simulink model "roachf_1024_bao"  (Simulink 7.5)
settings: Solver=ode45  StartTime=0.0  StopTime=10.0  RelTol=1e-3
undefined symbols (not defined in the file or in its folder): Down, quant, Up
libraries: xbsIndex_r4 x1081, xps_library x49, casper_library_misc x17, casper_library_delays x9, casper_library_sources x4, xbsReplacements_r4 x4, xrbsControl_r4 x1
(part 2 of 11)

== system roachf_1024_bao/status ==
  Concat : xbsIndex_r4/Concat  num_inputs=8  dbl_ovrd=off  block_type=concat
  Concat1 : xbsIndex_r4/Concat  num_inputs=8  dbl_ovrd=off  block_type=concat
  Constant1 : xbsIndex_r4/Constant  const=0  gui_display_data_type=Fixed-point  arith_type=Unsigned  n_bits=25  bin_pt=0  preci_type=Single  exp_width=8  frac_width=24  explicit_period=on  period=1  equ=P=C  opselect=C  inp2=PCIN>>17  opr=+  inp1=P  carry=CIN  dbl_ovrd=off  block_type=constant
      settings: block_version=11.4
  Constant2 : xbsIndex_r4/Constant  const=0  gui_display_data_type=Fixed-point  arith_type=Unsigned  n_bits=25  bin_pt=0  preci_type=Single  exp_width=8  frac_width=24  explicit_period=on  period=1  equ=P=C  opselect=C  inp2=PCIN>>17  opr=+  inp1=P  carry=CIN  dbl_ovrd=off  block_type=constant
      settings: block_version=11.4
  Counter1 : xbsIndex_r4/Counter  cnt_type=Free Running  cnt_to=Inf  operation=Up  start_count=0  cnt_by_val=1  arith_type=Unsigned  n_bits=32  bin_pt=0  load_pin=off  rst=on  en=on  explicit_period=on  period=1  dbl_ovrd=off  use_behavioral_HDL=off  implementation=Fabric  block_type=counter
  Counter2 : xbsIndex_r4/Counter  cnt_type=Free Running  cnt_to=Inf  operation=Up  start_count=0  cnt_by_val=1  arith_type=Unsigned  n_bits=32  bin_pt=0  load_pin=off  rst=on  en=on  explicit_period=on  period=1  dbl_ovrd=off  use_behavioral_HDL=off  implementation=Fabric  block_type=counter
  Counter3 : xbsIndex_r4/Counter  cnt_type=Free Running  cnt_to=Inf  operation=Up  start_count=0  cnt_by_val=1  arith_type=Unsigned  n_bits=32  bin_pt=0  load_pin=off  rst=on  en=on  explicit_period=on  period=1  dbl_ovrd=off  use_behavioral_HDL=off  implementation=Fabric  block_type=counter
  gbe_gpu : xps_library/software register  Tag=xps:sw_reg  SystemSampleTime=-1  io_dir=To Processor  arith_type=Unsigned  bitwidth=32  bin_pt=0  sample_period=1  gw_name=roachf_1024_bao_status_gbe_gpu_user_data_in
  gbe_sw : xps_library/software register  Tag=xps:sw_reg  SystemSampleTime=-1  io_dir=To Processor  arith_type=Unsigned  bitwidth=32  bin_pt=0  sample_period=1  gw_name=roachf_1024_bao_status_gbe_sw_user_data_in
  swgbe_bframe : xps_library/software register  Tag=xps:sw_reg  SystemSampleTime=-1  io_dir=To Processor  arith_type=Unsigned  bitwidth=32  bin_pt=0  sample_period=1  gw_name=roachf_1024_bao_status_swgbe_bframe_user_data_in
      link override convert: arith_type=Unsigned  n_bits=32  bin_pt=0
  swgbe_oflow : xps_library/software register  Tag=xps:sw_reg  SystemSampleTime=-1  io_dir=To Processor  arith_type=Unsigned  bitwidth=32  bin_pt=0  sample_period=1  gw_name=roachf_1024_bao_status_swgbe_oflow_user_data_in
      link override convert: arith_type=Unsigned  n_bits=32  bin_pt=0
  swgbe_orun : xps_library/software register  Tag=xps:sw_reg  SystemSampleTime=-1  io_dir=To Processor  arith_type=Unsigned  bitwidth=32  bin_pt=0  sample_period=1  gw_name=roachf_1024_bao_status_swgbe_orun_user_data_in
      link override convert: arith_type=Unsigned  n_bits=32  bin_pt=0
  wires:
  Concat/1 -> gbe_sw/1
  Constant1/1 -> Concat/1
  [gbe_sw_led_up] -> Concat/2
  [gbe_sw_led_rx] -> Concat/3
  [gbe_sw_led_tx] -> Concat/4
  [gbe_sw_tx_afull] -> Concat/5
  [gbe_sw_tx_oflow] -> Concat/6
  [gbe_sw_rx_bfr] -> Concat/7
  [gbe_sw_rx_orun] -> Concat/8
  Concat1/1 -> gbe_gpu/1
  Constant2/1 -> Concat1/1
  [gbe_gpu_led_up] -> Concat1/2
  [gbe_gpu_led_rx] -> Concat1/3
  [gbe_gpu_led_tx] -> Concat1/4
  [gbe_gpu_tx_ack] -> Concat1/5
  [gbe_gpu_rx_valid] -> Concat1/6
  [gbe_gpu_rx_eof] -> Concat1/7
  [gbe_gpu_rx_eof] -> Concat1/8
  Counter2/1 -> swgbe_bframe/1
  [gbe_sw_rx_bfr] -> Counter2/2
  [cnt_rst] -> Counter2/1
  Counter1/1 -> swgbe_orun/1
  [gbe_sw_rx_orun] -> Counter1/2
  [cnt_rst] -> Counter1/1
  Counter3/1 -> swgbe_oflow/1
  [gbe_sw_tx_oflow] -> Counter3/2
  [cnt_rst] -> Counter3/1

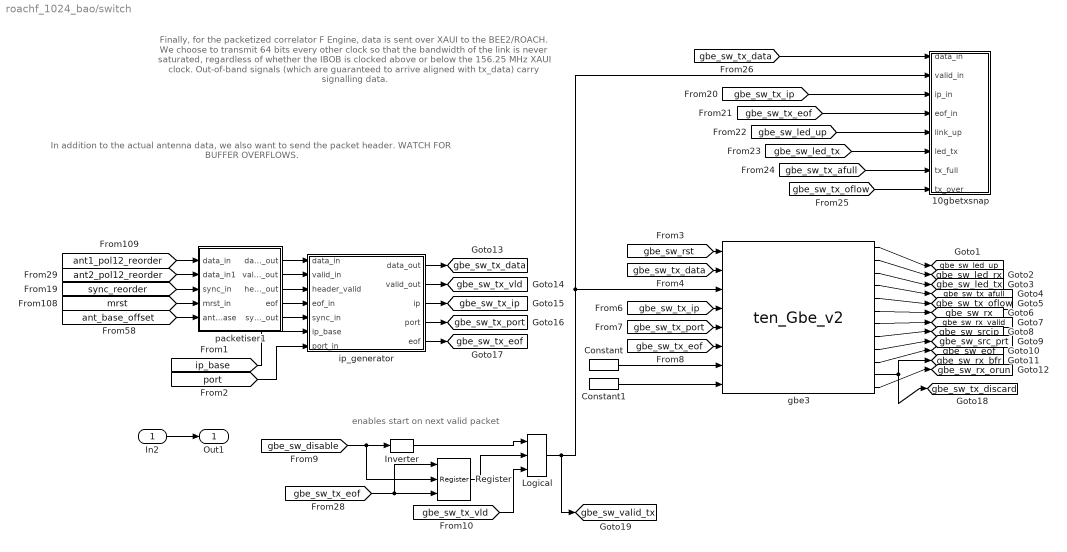
== system roachf_1024_bao/switch ==
  note: Finally, for the packetized correlator F Engine, data is sent over
      | XAUI to the BEE2/ROACH.  We choose to transmit 64 bits every other clock
      | so that the bandwidth of the link is never saturated, regardless of whether
      | the IBOB is clocked above or below the 156.25 MHz XAUI clock.
      | Out-of-band signals (which are guaranteed to arrive aligned with
      | tx_data) carry signalling data.
  note: In addition to the actual antenna data,
      | we also want to send the packet header.
      | WATCH FOR BUFFER OVERFLOWS.
  note: enables start on next valid packet
  In2 : Inport
  10gbetxsnap : Subsystem  mask{nsamples=10}
      mask prompts: nsamples "Number of samples (2^?)"
  Constant : xbsIndex_r4/Constant  const=1  gui_display_data_type=Fixed-point  arith_type=Boolean  n_bits=16  bin_pt=14  preci_type=Single  exp_width=8  frac_width=24  explicit_period=on  period=1  equ=P=C  opselect=C  inp2=PCIN>>17  opr=+  inp1=P  carry=CIN  dbl_ovrd=off  block_type=constant
      settings: block_version=11.4
  Constant1 : xbsIndex_r4/Constant  const=0  gui_display_data_type=Fixed-point  arith_type=Boolean  n_bits=16  bin_pt=14  preci_type=Single  exp_width=8  frac_width=24  explicit_period=on  period=1  equ=P=C  opselect=C  inp2=PCIN>>17  opr=+  inp1=P  carry=CIN  dbl_ovrd=off  block_type=constant
      settings: block_version=11.4
  Inverter : xbsIndex_r4/Inverter  en=off  latency=0  dbl_ovrd=off  block_type=inv
      settings: block_version=11.4
  Logical : xbsIndex_r4/Logical  logical_function=AND  inputs=3  en=off  latency=0  precision=Full  arith_type=Unsigned  n_bits=16  bin_pt=0  align_bp=on  dbl_ovrd=off  block_type=logical
      settings: block_version=11.4
  Register : xbsIndex_r4/Register  init=0  rst=on  en=on  dbl_ovrd=off  block_type=register
  gbe3 : xps_library/ten_Gbe_v2  Tag=xps:tengbe_v2  SystemSampleTime=-1  port=3  rx_dist_ram=off  large_frames=on  show_param=off  pre_emph=3  swing=800  fab_en=off  fab_mac=hex2dec('123456780000')  fab_ip=192*(2^24) + 168*(2^16) + 5*(2^8) + 20*(2^0)  fab_udp=10000  fab_gate=1  cpu_rx_en=on  cpu_tx_en=on
  ip_generator : Subsystem
  packetiser1 : Subsystem  mask{nwrd_bits=10, ant_bits=1, nSpec=4, nXeng=3, nChan=10}
      mask prompts: nwrd_bits "Payload length: (in 64bit words) (2^n)"; ant_bits "Number of antennas on this link (2^n)"; nSpec "Number of spectra(time samples) to acc. (2^?)"; nXeng "Number of Xengines total (2^?)"; nChan "Number of Channels in a spectra(2^?)"
      mask help: Wideband packetiser. Package 32 bit data into 64 bits and identify data as coming from antenna 0 or 1.
  Out1 : Outport
  tag scope: gbe_sw_eof=global, gbe_sw_led_rx=global, gbe_sw_led_tx=global, gbe_sw_led_up=global, gbe_sw_rx=global, gbe_sw_rx_bfr=global, gbe_sw_rx_orun=global, gbe_sw_rx_valid=global, gbe_sw_src_prt=global, gbe_sw_srcip=global, gbe_sw_tx_afull=global, gbe_sw_tx_data=global, gbe_sw_tx_discard=global, gbe_sw_tx_eof=global, gbe_sw_tx_ip=global, gbe_sw_tx_oflow=global, gbe_sw_tx_port=global, gbe_sw_tx_vld=global, gbe_sw_valid_tx=global
  wires:
  [sync_reorder] -> packetiser1/3(sync_in)
  [mrst] -> packetiser1/4(mrst_in)
  [ant1_pol12_reorder] -> packetiser1/1(data_in)
  [ant_base_offset] -> packetiser1/5(ant_base)
  packetiser1/5(sync_out) -> ip_generator/5(sync_in)
  packetiser1/4(eof) -> ip_generator/4(eof_in)
  packetiser1/3(header_out) -> ip_generator/3(header_valid)
  packetiser1/2(valid_out) -> ip_generator/2(valid_in)
  packetiser1/1(data_out) -> ip_generator/1(data_in)
  In2/1 -> Out1/1
  [ip_base] -> ip_generator/6(ip_base)
  [port] -> ip_generator/7(port_in)
  [gbe_sw_rst] -> gbe3/1
  gbe3/1 -> [gbe_sw_led_up]
  gbe3/2 -> [gbe_sw_led_rx]
  gbe3/3 -> [gbe_sw_led_tx]
  gbe3/4 -> [gbe_sw_tx_afull]
  gbe3/5 -> [gbe_sw_tx_oflow]
  gbe3/6 -> [gbe_sw_rx]
  gbe3/7 -> [gbe_sw_rx_valid]
  gbe3/8 -> [gbe_sw_srcip]
  gbe3/9 -> [gbe_sw_src_prt]
  gbe3/10 -> [gbe_sw_eof]
  gbe3/11 -> [gbe_sw_rx_bfr], [gbe_sw_tx_discard]
  gbe3/12 -> [gbe_sw_rx_orun]
  ip_generator/1(data_out) -> [gbe_sw_tx_data]
  ip_generator/2(valid_out) -> [gbe_sw_tx_vld]
  ip_generator/3(ip) -> [gbe_sw_tx_ip]
  ip_generator/4(port) -> [gbe_sw_tx_port]
  ip_generator/5(eof) -> [gbe_sw_tx_eof]
  Constant/1 -> gbe3/7
  Constant1/1 -> gbe3/8
  [gbe_sw_tx_data] -> gbe3/2
  Logical/1 -> gbe3/3, 10gbetxsnap/2(valid_in), [gbe_sw_valid_tx]
  [gbe_sw_tx_ip] -> gbe3/4
  [gbe_sw_tx_port] -> gbe3/5
  [gbe_sw_tx_eof] -> gbe3/6
  [gbe_sw_disable] -> Inverter/1, Register/2
  Inverter/1 -> Logical/1
  [gbe_sw_led_tx] -> 10gbetxsnap/6(led_tx)
  [gbe_sw_tx_afull] -> 10gbetxsnap/7(tx_full)
  [gbe_sw_tx_oflow] -> 10gbetxsnap/8(tx_over)
  [gbe_sw_led_up] -> 10gbetxsnap/5(link_up)
  [gbe_sw_tx_eof] -> 10gbetxsnap/4(eof_in)
  [gbe_sw_tx_data] -> 10gbetxsnap/1(data_in)
  [gbe_sw_tx_ip] -> 10gbetxsnap/3(ip_in)
  Register/1 -> Logical/2
  [gbe_sw_tx_eof] -> Register/3, Register/1
  [gbe_sw_tx_vld] -> Logical/3
  [ant2_pol12_reorder] -> packetiser1/2(data_in1)

== system roachf_1024_bao/transpose ==
  note: A matrix transpose is performed in SRAM so that 128 samples of frequency
      | channel 0 are output, followed by 128 samples of channel 1, and so forth.
      | These blocks of samples for a single channel are turned into 10 GbE packets
      | on the X engine, and are then routed through a swittch.  "one_ant_a_time"
      | outputs 128 samples for channel 0 (both polarizations) of one antenna,
      | and then 128 samples for channel 0 of the other antenna, followed by
      | channel 1 of the first antenna, and so on.  This allows the X engine design to
      | pass data directly from the XAUI into a packet containing 128 time samples
      | for 1 frequency from 1 antenna.
  note: Currently "dbuf_ct_sram" double-buffers data (meaning it writes data
      | into one buffer, while reading data out in the desired order from another
      | buffer.  Look into QDR or bigger BRAMS to increas number of channels.
  note: A matrix transpose and reorder is performed in Shared BRAMS.
      | Currently, 4 time samples of frequency%16 are output. for #channels = 2048
      | 128 channels (the channels to be sent to one xengine, in order 0,16,32,...for xengine0.
      | ch#1,17,33... for xeng1. etc..)
      | That is ch(mod16) = i gets sent to xengine i (wherever it maybe located).
  note: b={a[13],a[9:8],a[7:0],a[12:10]}
  note: b={a[13],a[9:8],a[0],a[12:10],a[7:1]}
  note: will be getting rid of 16 channels instead of 8.
  note: b = {a[12],a[8:5],a[11:1],[4:0]}
  note: reshape(reshape([0:511],8,64)',1,512)
  note: as of jun27
  note: as of jun27
  In1 : Inport
  BitBasher : xbsIndex_r4/BitBasher  bitexpr=|  display_expr=off  sr_1=1  arith_type1=Unsigned  bin_pt1=0  sr_2=2  arith_type2=Unsigned  bin_pt2=0  sr_3=3  arith_type3=Unsigned  bin_pt3=0  sr_4=4  arith_type4=Unsigned  bin_pt4=0  dbl_ovrd=off  block_type=bitbasher
      | <!DOCTYPE HTML PUBLIC "-//W3C//DTD HTML 4.0//EN" "http://www.w3.org/TR/REC-html40/strict.dtd">
      | <html><head><meta name="qrichtext" content="1" /><style type="text/css">
      | p, li { white-space: pre-wrap; }
      | </style></head><body style=" font-family:'Sans'; font-size:10pt; font-weight:400; font-style:normal;">
      | <p style=" margin-top:12px; margin-bottom:12px; margin-left:0px; margin-right:0px; -qt-block-indent:0; text-indent:0px;"><span style=" font-family:'MS Shell Dlg'; font-size:8pt;">even = {din[55:48],din[39:32],din[23:16],din[7:0]}<br />odd = {din[63:56],din[47:40],din[31:24],din[15:8]}</span></p></body></html>
  Constant : xbsIndex_r4/Constant  const=1  gui_display_data_type=Boolean  arith_type=Boolean  n_bits=16  bin_pt=14  preci_type=Single  exp_width=8  frac_width=24  explicit_period=on  period=1  equ=P=C  opselect=C  inp2=PCIN>>17  opr=+  inp1=P  carry=CIN  dbl_ovrd=off  block_type=constant
  Constant1 : xbsIndex_r4/Constant  const=1  gui_display_data_type=Boolean  arith_type=Boolean  n_bits=16  bin_pt=14  preci_type=Single  exp_width=8  frac_width=24  explicit_period=on  period=1  equ=P=C  opselect=C  inp2=PCIN>>17  opr=+  inp1=P  carry=CIN  dbl_ovrd=off  block_type=constant
  Delay1 : Subsystem  AncestorBlock=casper_library/Delays/pipeline  mask(pipeline){latency=1}
      mask help:
      | An explicitly laid-out delay line to avoid mapping to SRL16s
      | for use in pipelining to help achieve timing closure.
      mask init:
      | pipeline_init(gcb, 'latency', latency);
      mask Display:
      | port_label('input', 1, 'd');
      | port_label('output', 1, 'q');
      | disp(['Z^-', num2str(latency)]);
  Delay2 : Subsystem  AncestorBlock=casper_library/Delays/pipeline  mask(pipeline){latency=1}
      mask help:
      | An explicitly laid-out delay line to avoid mapping to SRL16s
      | for use in pipelining to help achieve timing closure.
      mask init:
      | pipeline_init(gcb, 'latency', latency);
      mask Display:
      | port_label('input', 1, 'd');
      | port_label('output', 1, 'q');
      | disp(['Z^-', num2str(latency)]);
  Delay3 : Subsystem  AncestorBlock=casper_library/Delays/pipeline  mask(pipeline){latency=1}
      mask help:
      | An explicitly laid-out delay line to avoid mapping to SRL16s
      | for use in pipelining to help achieve timing closure.
      mask init:
      | pipeline_init(gcb, 'latency', latency);
      mask Display:
      | port_label('input', 1, 'd');
      | port_label('output', 1, 'q');
      | disp(['Z^-', num2str(latency)]);
  Delay5 : Subsystem  AncestorBlock=casper_library/Delays/pipeline  mask(pipeline){latency=1}
      mask help:
      | An explicitly laid-out delay line to avoid mapping to SRL16s
      | for use in pipelining to help achieve timing closure.
      mask init:
      | pipeline_init(gcb, 'latency', latency);
      mask Display:
      | port_label('input', 1, 'd');
      | port_label('output', 1, 'q');
      | disp(['Z^-', num2str(latency)]);
  Delay79 : Subsystem  AncestorBlock=casper_library/Delays/pipeline  mask(pipeline){latency=1}
      mask help:
      | An explicitly laid-out delay line to avoid mapping to SRL16s
      | for use in pipelining to help achieve timing closure.
      mask init:
      | pipeline_init(gcb, 'latency', latency);
      mask Display:
      | port_label('input', 1, 'd');
      | port_label('output', 1, 'q');
      | disp(['Z^-', num2str(latency)]);
  qdr_reorder : Subsystem  mask{bitexp=b={a[12],a[8:5],a[11:9],a[4:0]}, len=10, numspec=4}
      mask prompts: bitexp "bit bash expr"; len "FFT Length (2^?)"; numspec "Time Samples (2^?)"
      mask init:
      | bblk = [gcb, '/BitBasher']
      | c = bitexp
      | set_param(bblk, 'bitexpr', c)
  qdr_reorder1 : Subsystem  mask{bitexp=b={a[12],a[8:5],a[11:9],a[4:0]}, len=10, numspec=4}
      mask prompts: bitexp "bit bash expr"; len "FFT Length (2^?)"; numspec "Time Samples (2^?)"
      mask init:
      | bblk = [gcb, '/BitBasher']
      | c = bitexp
      | set_param(bblk, 'bitexpr', c)
  reorder : Subsystem  AncestorBlock=casper_library_reorder/reorder  mask(reorder){map=getfield( getfield( get_param( gcb,'UserData' ), 'parameters'),'map'), n_inputs=1, bram_latency=1, map_latency=1, double_buffer=0, bram_map=off}
      mask prompts: map "Output Order:"; n_inputs "Number of inputs"; bram_latency "BRAM Latency"; map_latency "Map Latency"; double_buffer "Double Buffer"; bram_map "Use BlockRAM for Map"
      mask init:
      | reorder_init(gcb, ...
      |     'map', map, ...
      |     'n_inputs', n_inputs, ...
      |     'bram_latency', bram_latency, ...
      |     'map_latency', map_latency, ...
      |     'double_buffer', double_buffer, ...
      |     'bram_map', bram_map);
      settings: AttributesFormatString=order=3
      mask Help: eval('xlWeb(''http://casper.berkeley.edu/wiki/Reorder'')')
  reorder1 : Subsystem  AncestorBlock=casper_library_reorder/reorder  mask(reorder){map=getfield( getfield( get_param( gcb,'UserData' ), 'parameters'),'map'), n_inputs=1, bram_latency=1, map_latency=1, double_buffer=0, bram_map=off}
      mask prompts: map "Output Order:"; n_inputs "Number of inputs"; bram_latency "BRAM Latency"; map_latency "Map Latency"; double_buffer "Double Buffer"; bram_map "Use BlockRAM for Map"
      mask init: same as roachf_1024_bao/transpose/reorder
      settings: AttributesFormatString=order=3
      mask Help: eval('xlWeb(''http://casper.berkeley.edu/wiki/Reorder'')')
  Out1 : Outport
  tag scope: ant1_pol12_reorder=global, ant2_pol12_reorder=global, sync_reorder=global
  wires:
  [eq_out] -> Delay3/1(d)
  [sync_rnd] -> Delay2/1(d)
  In1/1 -> Out1/1
  Delay79/1(q) -> [ant1_pol12_reorder]
  Delay1/1(q) -> [sync_reorder]
  qdr_reorder/1(dataout) -> Delay79/1(d)
  qdr_reorder/2(syncout) -> Delay1/1(d)
  Delay5/1(q) -> [ant2_pol12_reorder]
  qdr_reorder1/1(dataout) -> Delay5/1(d)
  Delay3/1(q) -> BitBasher/1
  Constant/1 -> reorder/2(en)
  BitBasher/1 -> reorder/3(din0)
  Delay2/1(q) -> reorder/1(sync), reorder1/1(sync)
  reorder/1(sync_out) -> qdr_reorder/2(syncin)
  reorder/3(dout0) -> qdr_reorder/1(datain)
  BitBasher/2 -> reorder1/3(din0)
  Constant1/1 -> reorder1/2(en)
  reorder1/3(dout0) -> qdr_reorder1/1(datain)
  reorder1/1(sync_out) -> qdr_reorder1/2(syncin)

== system roachf_1024_bao/ADC's/pol_pack0 ==
  In1 : Inport
  In2 : Inport  Port=2
  In3 : Inport  Port=3
  In4 : Inport  Port=4
  Concat3 : xbsIndex_r4/Concat  num_inputs=4  dbl_ovrd=off  block_type=concat
      settings: block_version=10.1.3
  Reinterpret{4..7} (4 alike) : xbsIndex_r4/Reinterpret  force_arith_type=on  arith_type=Unsigned  force_bin_pt=on  bin_pt=0  block_type=reinterpret
      settings: infoedit="Changes signal type without altering the binary representation.   You can changed the signal between signed and unsigned, and relocate the binary point.<P><P>Hardware notes: In hardware this block costs nothing.<P><P>Example:  Suppose the input is 6 bits wide, signed, with 2 fractional bits, and the output is forced to unsigned with 0 fractional bits.  Then an input of -2.0 (1110.00 in binary 2's complement) becomes an output of 56 (111000 in binary)."  block_version=10.1.3
  Out1 : Outport
  wires:
  In4/1 -> Reinterpret7/1
  In3/1 -> Reinterpret6/1
  Concat3/1 -> Out1/1
  In2/1 -> Reinterpret5/1
  In1/1 -> Reinterpret4/1
  Reinterpret7/1 -> Concat3/4
  Reinterpret6/1 -> Concat3/3
  Reinterpret5/1 -> Concat3/2
  Reinterpret4/1 -> Concat3/1

== system roachf_1024_bao/ADC's/pol_pack1 ==
  In1 : Inport
  In2 : Inport  Port=2
  In3 : Inport  Port=3
  In4 : Inport  Port=4
  Concat3 : xbsIndex_r4/Concat  num_inputs=4  dbl_ovrd=off  block_type=concat
      settings: block_version=10.1.3
  Reinterpret{4..7} (4 alike) : xbsIndex_r4/Reinterpret  force_arith_type=on  arith_type=Unsigned  force_bin_pt=on  bin_pt=0  block_type=reinterpret
      settings: infoedit="Changes signal type without altering the binary representation.   You can changed the signal between signed and unsigned, and relocate the binary point.<P><P>Hardware notes: In hardware this block costs nothing.<P><P>Example:  Suppose the input is 6 bits wide, signed, with 2 fractional bits, and the output is forced to unsigned with 0 fractional bits.  Then an input of -2.0 (1110.00 in binary 2's complement) becomes an output of 56 (111000 in binary)."  block_version=10.1.3
  Out1 : Outport
  wires:
  Reinterpret4/1 -> Concat3/1
  Reinterpret5/1 -> Concat3/2
  Reinterpret6/1 -> Concat3/3
  Reinterpret7/1 -> Concat3/4
  In1/1 -> Reinterpret4/1
  In2/1 -> Reinterpret5/1
  Concat3/1 -> Out1/1
  In3/1 -> Reinterpret6/1
  In4/1 -> Reinterpret7/1

== system roachf_1024_bao/ADC's/pol_pack2 ==
  In1 : Inport
  In2 : Inport  Port=2
  In3 : Inport  Port=3
  In4 : Inport  Port=4
  Concat3 : xbsIndex_r4/Concat  num_inputs=4  dbl_ovrd=off  block_type=concat
      settings: block_version=10.1.3
  Reinterpret{4..7} (4 alike) : xbsIndex_r4/Reinterpret  force_arith_type=on  arith_type=Unsigned  force_bin_pt=on  bin_pt=0  block_type=reinterpret
      settings: infoedit="Changes signal type without altering the binary representation.   You can changed the signal between signed and unsigned, and relocate the binary point.<P><P>Hardware notes: In hardware this block costs nothing.<P><P>Example:  Suppose the input is 6 bits wide, signed, with 2 fractional bits, and the output is forced to unsigned with 0 fractional bits.  Then an input of -2.0 (1110.00 in binary 2's complement) becomes an output of 56 (111000 in binary)."  block_version=10.1.3
  Out1 : Outport
  wires:
  Reinterpret4/1 -> Concat3/1
  Reinterpret5/1 -> Concat3/2
  Reinterpret6/1 -> Concat3/3
  Reinterpret7/1 -> Concat3/4
  In1/1 -> Reinterpret4/1
  In2/1 -> Reinterpret5/1
  Concat3/1 -> Out1/1
  In3/1 -> Reinterpret6/1
  In4/1 -> Reinterpret7/1

== system roachf_1024_bao/ADC's/pol_pack3 ==
  In1 : Inport
  In2 : Inport  Port=2
  In3 : Inport  Port=3
  In4 : Inport  Port=4
  Concat3 : xbsIndex_r4/Concat  num_inputs=4  dbl_ovrd=off  block_type=concat
      settings: block_version=10.1.3
  Reinterpret{4..7} (4 alike) : xbsIndex_r4/Reinterpret  force_arith_type=on  arith_type=Unsigned  force_bin_pt=on  bin_pt=0  block_type=reinterpret
      settings: infoedit="Changes signal type without altering the binary representation.   You can changed the signal between signed and unsigned, and relocate the binary point.<P><P>Hardware notes: In hardware this block costs nothing.<P><P>Example:  Suppose the input is 6 bits wide, signed, with 2 fractional bits, and the output is forced to unsigned with 0 fractional bits.  Then an input of -2.0 (1110.00 in binary 2's complement) becomes an output of 56 (111000 in binary)."  block_version=10.1.3
  Out1 : Outport
  wires:
  In4/1 -> Reinterpret7/1
  In3/1 -> Reinterpret6/1
  Concat3/1 -> Out1/1
  In2/1 -> Reinterpret5/1
  In1/1 -> Reinterpret4/1
  Reinterpret7/1 -> Concat3/4
  Reinterpret6/1 -> Concat3/3
  Reinterpret5/1 -> Concat3/2
  Reinterpret4/1 -> Concat3/1

== system roachf_1024_bao/EQ/quant0 ==
  sync : Inport
  din0 : Inport  Port=2
  din1 : Inport  Port=3
  Constant19 : Constant  Value=0  OutDataType=sfix(16)  OutScaling=2^0
  Constant45 : Constant  Value=0  OutDataType=sfix(16)  OutScaling=2^0
  Convert : xbsIndex_r4/Convert  gui_display_data_type=Fixed-point  arith_type=Unsigned  n_bits=18  bin_pt=3  float_type=Single  exp_bits=8  fraction_bits=24  quantization=Truncate  overflow=Wrap  en=off  latency=0  dbl_ovrd=off  pipeline=off  block_type=convert
      settings: block_version=10.1.3
  Convert1 : xbsIndex_r4/Convert  gui_display_data_type=Fixed-point  arith_type=Unsigned  n_bits=18  bin_pt=3  float_type=Single  exp_bits=8  fraction_bits=24  quantization=Truncate  overflow=Wrap  en=off  latency=0  dbl_ovrd=off  pipeline=off  block_type=convert
      settings: block_version=10.1.3
  Convert2 : xbsIndex_r4/Convert  gui_display_data_type=Fixed-point  arith_type=Unsigned  n_bits=18  bin_pt=3  float_type=Single  exp_bits=8  fraction_bits=24  quantization=Truncate  overflow=Wrap  en=off  latency=0  dbl_ovrd=off  pipeline=off  block_type=convert
      settings: block_version=10.1.3
  Delay{1..3,5,15,17} (6 alike) : xbsIndex_r4/Delay  rst=off  infoeditControl=Selection of Reset will increase slice count due to use of real FFs and instead of SRLs  en=off  latency=1  dbl_ovrd=off  reg_retiming=on  block_type=delay
      settings: xl_area=[0, 0, 0, 0, 0, 0, 0]
  Delay18 : xbsIndex_r4/Delay  rst=off  infoeditControl=Selection of Reset will increase slice count due to use of real FFs and instead of SRLs  en=off  latency=1  dbl_ovrd=off  reg_retiming=off  block_type=delay
      settings: xl_area=[0, 0, 0, 0, 0, 0, 0]
  Delay19 : xbsIndex_r4/Delay  rst=off  infoeditControl=Selection of Reset will increase slice count due to use of real FFs and instead of SRLs  en=off  latency=7  dbl_ovrd=off  reg_retiming=off  block_type=delay
      settings: xl_area=[0, 0, 0, 0, 0, 0, 0]
  Delay25 : xbsIndex_r4/Delay  rst=off  infoeditControl=Selection of Reset will increase slice count due to use of real FFs and instead of SRLs  en=off  latency=1  dbl_ovrd=off  reg_retiming=off  block_type=delay
      settings: xl_area=[0, 0, 0, 0, 0, 0, 0]
  Logical5 : xbsIndex_r4/Logical  logical_function=OR  inputs=2  en=off  latency=0  precision=Full  arith_type=Unsigned  n_bits=8  bin_pt=2  align_bp=on  dbl_ovrd=off  block_type=logical
      settings: xl_area=[0, 0, 0, 0, 0, 0, 0]
  Slice11 : xbsIndex_r4/Slice  nbits=18  boolean_output=off  mode=Lower Bit Location + Width  bit1=0  base1=MSB of Input  bit0=0  base0=LSB of Input  dbl_ovrd=off  block_type=slice
      settings: infoedit="Extracts a given range of bits from each input sample and presents it at the output.  The output type is ordinarily unsigned with binary point at zero, but can be Boolean when the slice is one bit wide.<P><P>Hardware notes: In hardware this block costs nothing."  block_version=10.1.3
  Slice14 : xbsIndex_r4/Slice  nbits=18  boolean_output=off  mode=Lower Bit Location + Width  bit1=0  base1=MSB of Input  bit0=18  base0=LSB of Input  dbl_ovrd=off  block_type=slice
      settings: infoedit="Extracts a given range of bits from each input sample and presents it at the output.  The output type is ordinarily unsigned with binary point at zero, but can be Boolean when the slice is one bit wide.<P><P>Hardware notes: In hardware this block costs nothing."  block_version=10.1.3
  Slice40 : xbsIndex_r4/Slice  nbits=18  boolean_output=off  mode=Lower Bit Location + Width  bit1=0  base1=MSB of Input  bit0=0  base0=LSB of Input  dbl_ovrd=off  block_type=slice
      settings: infoedit="Extracts a given range of bits from each input sample and presents it at the output.  The output type is ordinarily unsigned with binary point at zero, but can be Boolean when the slice is one bit wide.<P><P>Hardware notes: In hardware this block costs nothing."  block_version=10.1.3
  Slice7 : xbsIndex_r4/Slice  nbits=10  boolean_output=off  mode=Lower Bit Location + Width  bit1=0  base1=MSB of Input  bit0=0  base0=LSB of Input  dbl_ovrd=off  block_type=slice
      settings: infoedit="Extracts a given range of bits from each input sample and presents it at the output.  The output type is ordinarily unsigned with binary point at zero, but can be Boolean when the slice is one bit wide.<P><P>Hardware notes: In hardware this block costs nothing."  block_version=10.1.3
  addr : xps_library/software register  Tag=xps:sw_reg  SystemSampleTime=-1  io_dir=From Processor  arith_type=Unsigned  bitwidth=32  bin_pt=0  sample_period=1  gw_name=roachf_1024_bao_EQ_quant0_addr_user_data_out
      link override baopoco_quant0_addr_user_data_out: arith_type=Unsigned  n_bits=32  bin_pt=0  period=1
      link override poco_mod_1024_eq_scale0_user_data_out: arith_type=Unsigned  n_bits=32  bin_pt=0  period=1
      link override poco_mod_1024_no_fd_eq_scale0_user_data_out: arith_type=Unsigned  n_bits=32  bin_pt=0  period=1
      link override poco_mod_eq_scale_user_data_out: arith_type=Unsigned  n_bits=32  bin_pt=0  period=1
      link override poco_red_cd_ld_time_msb_user_data_out: arith_type=Unsigned  n_bits=32  bin_pt=0  period=1
      link override poco_red_fd_ld_time_msb_user_data_out: arith_type=Unsigned  n_bits=32  bin_pt=0  period=1
      link override poco_ref_roach_adc0_cd_ld_time_msb_user_data_out: arith_type=Unsigned  n_bits=32  bin_pt=0  period=1
      link override poco_ref_roach_reduced_adc0_cd_ld_time_msb_user_data_out: arith_type=Unsigned  n_bits=32  bin_pt=0  period=1
      link override poco_roach_red_adc0_cd_ld_time_msb_user_data_out: arith_type=Unsigned  n_bits=32  bin_pt=0  period=1
      link override poco_wide_10_r309_eq_scale0_user_data_out: arith_type=Unsigned  n_bits=32  bin_pt=0  period=1
      link override poco_wide_10_r310_quant0_addr_user_data_out: arith_type=Unsigned  n_bits=32  bin_pt=0  period=1
      link override poco_wide_10_r310_quant3_addr_user_data_out: arith_type=Unsigned  n_bits=32  bin_pt=0  period=1
  eq_store0 : Subsystem  mask{depth_bits=10, n_par=2}
      mask prompts: depth_bits "Number of channels (2^?)"; n_par "Number of parallel streams"
  gain : xps_library/software register  Tag=xps:sw_reg  SystemSampleTime=-1  io_dir=From Processor  arith_type=Unsigned  bitwidth=32  bin_pt=0  sample_period=1  gw_name=roachf_1024_bao_EQ_quant0_gain_user_data_out
      link override baopoco_quant0_gain_user_data_out: arith_type=Unsigned  n_bits=32  bin_pt=0  period=1
      link override poco_mod_1024_eq_scale0_user_data_out: arith_type=Unsigned  n_bits=32  bin_pt=0  period=1
      link override poco_mod_1024_no_fd_eq_scale0_user_data_out: arith_type=Unsigned  n_bits=32  bin_pt=0  period=1
      link override poco_mod_eq_scale_user_data_out: arith_type=Unsigned  n_bits=32  bin_pt=0  period=1
      link override poco_red_cd_ld_time_msb_user_data_out: arith_type=Unsigned  n_bits=32  bin_pt=0  period=1
      link override poco_red_fd_ld_time_msb_user_data_out: arith_type=Unsigned  n_bits=32  bin_pt=0  period=1
      link override poco_ref_roach_adc0_cd_ld_time_msb_user_data_out: arith_type=Unsigned  n_bits=32  bin_pt=0  period=1
      link override poco_ref_roach_reduced_adc0_cd_ld_time_msb_user_data_out: arith_type=Unsigned  n_bits=32  bin_pt=0  period=1
      link override poco_roach_red_adc0_cd_ld_time_msb_user_data_out: arith_type=Unsigned  n_bits=32  bin_pt=0  period=1
      link override poco_wide_10_r309_eq_scale0_user_data_out: arith_type=Unsigned  n_bits=32  bin_pt=0  period=1
      link override poco_wide_10_r310_quant0_gain_user_data_out: arith_type=Unsigned  n_bits=32  bin_pt=0  period=1
      link override poco_wide_10_r310_quant3_gain_user_data_out: arith_type=Unsigned  n_bits=32  bin_pt=0  period=1
  round1 : Subsystem  mask{n_bits=4}
      mask prompts: n_bits "Output Bitwidth"
  round2 : Subsystem  mask{n_bits=4}
      mask prompts: n_bits "Output Bitwidth"
  sync_out : Outport
  clip_out : Outport  Port=2
  dout0 : Outport  Port=3
  dout1 : Outport  Port=4
  wires:
  round1/2(clip) -> Logical5/1
  round2/2(clip) -> Logical5/2
  Constant45/1 -> gain/1
  gain/1 -> Slice40/1
  Slice40/1 -> Delay15/1
  Delay15/1 -> Convert/1
  Delay19/1 -> sync_out/1
  Convert/1 -> eq_store0/2(coeff)
  Slice14/1 -> Convert1/1
  Slice11/1 -> Convert2/1
  eq_store0/1(scale) -> Delay1/1
  Convert1/1 -> round1/2(scale)
  Convert2/1 -> round2/2(scale)
  Constant19/1 -> addr/1
  addr/1 -> Slice7/1
  Slice7/1 -> Delay17/1
  Delay17/1 -> eq_store0/3(coeff_addr)
  Delay18/1 -> Delay3/1
  Delay25/1 -> Delay2/1
  sync/1 -> eq_store0/1(sync), Delay19/1
  din0/1 -> Delay18/1
  round1/1(dout) -> dout0/1
  Logical5/1 -> Delay5/1
  din1/1 -> Delay25/1
  round2/1(dout) -> dout1/1
  Delay1/1 -> Slice11/1, Slice14/1
  Delay2/1 -> round2/1(din)
  Delay3/1 -> round1/1(din)
  Delay5/1 -> clip_out/1

== system roachf_1024_bao/EQ/quant1 ==
  sync : Inport
  din0 : Inport  Port=2
  din1 : Inport  Port=3
  Constant19 : Constant  Value=0  OutDataType=sfix(16)  OutScaling=2^0
  Constant45 : Constant  Value=0  OutDataType=sfix(16)  OutScaling=2^0
  Convert : xbsIndex_r4/Convert  gui_display_data_type=Fixed-point  arith_type=Unsigned  n_bits=18  bin_pt=3  float_type=Single  exp_bits=8  fraction_bits=24  quantization=Truncate  overflow=Wrap  en=off  latency=0  dbl_ovrd=off  pipeline=off  block_type=convert
      settings: block_version=10.1.3
  Convert1 : xbsIndex_r4/Convert  gui_display_data_type=Fixed-point  arith_type=Unsigned  n_bits=18  bin_pt=3  float_type=Single  exp_bits=8  fraction_bits=24  quantization=Truncate  overflow=Wrap  en=off  latency=0  dbl_ovrd=off  pipeline=off  block_type=convert
      settings: block_version=10.1.3
  Convert2 : xbsIndex_r4/Convert  gui_display_data_type=Fixed-point  arith_type=Unsigned  n_bits=18  bin_pt=3  float_type=Single  exp_bits=8  fraction_bits=24  quantization=Truncate  overflow=Wrap  en=off  latency=0  dbl_ovrd=off  pipeline=off  block_type=convert
      settings: block_version=10.1.3
  Delay{1..3,5,15,17} (6 alike) : xbsIndex_r4/Delay  rst=off  infoeditControl=Selection of Reset will increase slice count due to use of real FFs and instead of SRLs  en=off  latency=1  dbl_ovrd=off  reg_retiming=on  block_type=delay
      settings: xl_area=[0, 0, 0, 0, 0, 0, 0]
  Delay18 : xbsIndex_r4/Delay  rst=off  infoeditControl=Selection of Reset will increase slice count due to use of real FFs and instead of SRLs  en=off  latency=1  dbl_ovrd=off  reg_retiming=off  block_type=delay
      settings: xl_area=[0, 0, 0, 0, 0, 0, 0]
  Delay19 : xbsIndex_r4/Delay  rst=off  infoeditControl=Selection of Reset will increase slice count due to use of real FFs and instead of SRLs  en=off  latency=7  dbl_ovrd=off  reg_retiming=off  block_type=delay
      settings: xl_area=[0, 0, 0, 0, 0, 0, 0]
  Delay25 : xbsIndex_r4/Delay  rst=off  infoeditControl=Selection of Reset will increase slice count due to use of real FFs and instead of SRLs  en=off  latency=1  dbl_ovrd=off  reg_retiming=off  block_type=delay
      settings: xl_area=[0, 0, 0, 0, 0, 0, 0]
  Logical5 : xbsIndex_r4/Logical  logical_function=OR  inputs=2  en=off  latency=0  precision=Full  arith_type=Unsigned  n_bits=8  bin_pt=2  align_bp=on  dbl_ovrd=off  block_type=logical
      settings: xl_area=[0, 0, 0, 0, 0, 0, 0]
  Slice11 : xbsIndex_r4/Slice  nbits=18  boolean_output=off  mode=Lower Bit Location + Width  bit1=0  base1=MSB of Input  bit0=0  base0=LSB of Input  dbl_ovrd=off  block_type=slice
      settings: infoedit="Extracts a given range of bits from each input sample and presents it at the output.  The output type is ordinarily unsigned with binary point at zero, but can be Boolean when the slice is one bit wide.<P><P>Hardware notes: In hardware this block costs nothing."  block_version=10.1.3
  Slice14 : xbsIndex_r4/Slice  nbits=18  boolean_output=off  mode=Lower Bit Location + Width  bit1=0  base1=MSB of Input  bit0=18  base0=LSB of Input  dbl_ovrd=off  block_type=slice
      settings: infoedit="Extracts a given range of bits from each input sample and presents it at the output.  The output type is ordinarily unsigned with binary point at zero, but can be Boolean when the slice is one bit wide.<P><P>Hardware notes: In hardware this block costs nothing."  block_version=10.1.3
  Slice40 : xbsIndex_r4/Slice  nbits=18  boolean_output=off  mode=Lower Bit Location + Width  bit1=0  base1=MSB of Input  bit0=0  base0=LSB of Input  dbl_ovrd=off  block_type=slice
      settings: infoedit="Extracts a given range of bits from each input sample and presents it at the output.  The output type is ordinarily unsigned with binary point at zero, but can be Boolean when the slice is one bit wide.<P><P>Hardware notes: In hardware this block costs nothing."  block_version=10.1.3
  Slice7 : xbsIndex_r4/Slice  nbits=10  boolean_output=off  mode=Lower Bit Location + Width  bit1=0  base1=MSB of Input  bit0=0  base0=LSB of Input  dbl_ovrd=off  block_type=slice
      settings: infoedit="Extracts a given range of bits from each input sample and presents it at the output.  The output type is ordinarily unsigned with binary point at zero, but can be Boolean when the slice is one bit wide.<P><P>Hardware notes: In hardware this block costs nothing."  block_version=10.1.3
  addr : xps_library/software register  Tag=xps:sw_reg  SystemSampleTime=-1  io_dir=From Processor  arith_type=Unsigned  bitwidth=32  bin_pt=0  sample_period=1  gw_name=roachf_1024_bao_EQ_quant1_addr_user_data_out
      link override baopoco_quant0_addr_user_data_out: arith_type=Unsigned  n_bits=32  bin_pt=0  period=1
      link override poco_mod_1024_eq_scale0_user_data_out: arith_type=Unsigned  n_bits=32  bin_pt=0  period=1
      link override poco_mod_1024_no_fd_eq_scale0_user_data_out: arith_type=Unsigned  n_bits=32  bin_pt=0  period=1
      link override poco_mod_eq_scale_user_data_out: arith_type=Unsigned  n_bits=32  bin_pt=0  period=1
      link override poco_red_cd_ld_time_msb_user_data_out: arith_type=Unsigned  n_bits=32  bin_pt=0  period=1
      link override poco_red_fd_ld_time_msb_user_data_out: arith_type=Unsigned  n_bits=32  bin_pt=0  period=1
      link override poco_ref_roach_adc0_cd_ld_time_msb_user_data_out: arith_type=Unsigned  n_bits=32  bin_pt=0  period=1
      link override poco_ref_roach_reduced_adc0_cd_ld_time_msb_user_data_out: arith_type=Unsigned  n_bits=32  bin_pt=0  period=1
      link override poco_roach_red_adc0_cd_ld_time_msb_user_data_out: arith_type=Unsigned  n_bits=32  bin_pt=0  period=1
      link override poco_wide_10_r309_eq_scale0_user_data_out: arith_type=Unsigned  n_bits=32  bin_pt=0  period=1
      link override poco_wide_10_r310_quant0_addr_user_data_out: arith_type=Unsigned  n_bits=32  bin_pt=0  period=1
      link override poco_wide_10_r310_quant3_addr_user_data_out: arith_type=Unsigned  n_bits=32  bin_pt=0  period=1
  eq_store0 : Subsystem  mask{depth_bits=10, n_par=2}
      mask prompts: depth_bits "Number of channels (2^?)"; n_par "Number of parallel streams"
  gain : xps_library/software register  Tag=xps:sw_reg  SystemSampleTime=-1  io_dir=From Processor  arith_type=Unsigned  bitwidth=32  bin_pt=0  sample_period=1  gw_name=roachf_1024_bao_EQ_quant1_gain_user_data_out
      link override baopoco_quant0_gain_user_data_out: arith_type=Unsigned  n_bits=32  bin_pt=0  period=1
      link override poco_mod_1024_eq_scale0_user_data_out: arith_type=Unsigned  n_bits=32  bin_pt=0  period=1
      link override poco_mod_1024_no_fd_eq_scale0_user_data_out: arith_type=Unsigned  n_bits=32  bin_pt=0  period=1
      link override poco_mod_eq_scale_user_data_out: arith_type=Unsigned  n_bits=32  bin_pt=0  period=1
      link override poco_red_cd_ld_time_msb_user_data_out: arith_type=Unsigned  n_bits=32  bin_pt=0  period=1
      link override poco_red_fd_ld_time_msb_user_data_out: arith_type=Unsigned  n_bits=32  bin_pt=0  period=1
      link override poco_ref_roach_adc0_cd_ld_time_msb_user_data_out: arith_type=Unsigned  n_bits=32  bin_pt=0  period=1
      link override poco_ref_roach_reduced_adc0_cd_ld_time_msb_user_data_out: arith_type=Unsigned  n_bits=32  bin_pt=0  period=1
      link override poco_roach_red_adc0_cd_ld_time_msb_user_data_out: arith_type=Unsigned  n_bits=32  bin_pt=0  period=1
      link override poco_wide_10_r309_eq_scale0_user_data_out: arith_type=Unsigned  n_bits=32  bin_pt=0  period=1
      link override poco_wide_10_r310_quant0_gain_user_data_out: arith_type=Unsigned  n_bits=32  bin_pt=0  period=1
      link override poco_wide_10_r310_quant3_gain_user_data_out: arith_type=Unsigned  n_bits=32  bin_pt=0  period=1
  round1 : Subsystem  mask{n_bits=4}
      mask prompts: n_bits "Output Bitwidth"
  round2 : Subsystem  mask{n_bits=4}
      mask prompts: n_bits "Output Bitwidth"
  sync_out : Outport
  clip_out : Outport  Port=2
  dout0 : Outport  Port=3
  dout1 : Outport  Port=4
  wires:
  round1/2(clip) -> Logical5/1
  round2/2(clip) -> Logical5/2
  Constant45/1 -> gain/1
  gain/1 -> Slice40/1
  Slice40/1 -> Delay15/1
  Delay15/1 -> Convert/1
  Delay19/1 -> sync_out/1
  Convert/1 -> eq_store0/2(coeff)
  Slice14/1 -> Convert1/1
  Slice11/1 -> Convert2/1
  eq_store0/1(scale) -> Delay1/1
  Convert1/1 -> round1/2(scale)
  Convert2/1 -> round2/2(scale)
  Constant19/1 -> addr/1
  addr/1 -> Slice7/1
  Slice7/1 -> Delay17/1
  Delay17/1 -> eq_store0/3(coeff_addr)
  Delay18/1 -> Delay3/1
  Delay25/1 -> Delay2/1
  sync/1 -> eq_store0/1(sync), Delay19/1
  din0/1 -> Delay18/1
  round1/1(dout) -> dout0/1
  Logical5/1 -> Delay5/1
  din1/1 -> Delay25/1
  round2/1(dout) -> dout1/1
  Delay1/1 -> Slice11/1, Slice14/1
  Delay2/1 -> round2/1(din)
  Delay3/1 -> round1/1(din)
  Delay5/1 -> clip_out/1

== system roachf_1024_bao/EQ/quant2 ==
  sync : Inport
  din0 : Inport  Port=2
  din1 : Inport  Port=3
  Constant19 : Constant  Value=0  OutDataType=sfix(16)  OutScaling=2^0
  Constant45 : Constant  Value=0  OutDataType=sfix(16)  OutScaling=2^0
  Convert : xbsIndex_r4/Convert  gui_display_data_type=Fixed-point  arith_type=Unsigned  n_bits=18  bin_pt=3  float_type=Single  exp_bits=8  fraction_bits=24  quantization=Truncate  overflow=Wrap  en=off  latency=0  dbl_ovrd=off  pipeline=off  block_type=convert
      settings: block_version=10.1.3
  Convert1 : xbsIndex_r4/Convert  gui_display_data_type=Fixed-point  arith_type=Unsigned  n_bits=18  bin_pt=3  float_type=Single  exp_bits=8  fraction_bits=24  quantization=Truncate  overflow=Wrap  en=off  latency=0  dbl_ovrd=off  pipeline=off  block_type=convert
      settings: block_version=10.1.3
  Convert2 : xbsIndex_r4/Convert  gui_display_data_type=Fixed-point  arith_type=Unsigned  n_bits=18  bin_pt=3  float_type=Single  exp_bits=8  fraction_bits=24  quantization=Truncate  overflow=Wrap  en=off  latency=0  dbl_ovrd=off  pipeline=off  block_type=convert
      settings: block_version=10.1.3
  Delay{1..3,5,15,17} (6 alike) : xbsIndex_r4/Delay  rst=off  infoeditControl=Selection of Reset will increase slice count due to use of real FFs and instead of SRLs  en=off  latency=1  dbl_ovrd=off  reg_retiming=on  block_type=delay
      settings: xl_area=[0, 0, 0, 0, 0, 0, 0]
  Delay18 : xbsIndex_r4/Delay  rst=off  infoeditControl=Selection of Reset will increase slice count due to use of real FFs and instead of SRLs  en=off  latency=1  dbl_ovrd=off  reg_retiming=off  block_type=delay
      settings: xl_area=[0, 0, 0, 0, 0, 0, 0]
  Delay19 : xbsIndex_r4/Delay  rst=off  infoeditControl=Selection of Reset will increase slice count due to use of real FFs and instead of SRLs  en=off  latency=7  dbl_ovrd=off  reg_retiming=off  block_type=delay
      settings: xl_area=[0, 0, 0, 0, 0, 0, 0]
  Delay25 : xbsIndex_r4/Delay  rst=off  infoeditControl=Selection of Reset will increase slice count due to use of real FFs and instead of SRLs  en=off  latency=1  dbl_ovrd=off  reg_retiming=off  block_type=delay
      settings: xl_area=[0, 0, 0, 0, 0, 0, 0]
  Logical5 : xbsIndex_r4/Logical  logical_function=OR  inputs=2  en=off  latency=0  precision=Full  arith_type=Unsigned  n_bits=8  bin_pt=2  align_bp=on  dbl_ovrd=off  block_type=logical
      settings: xl_area=[0, 0, 0, 0, 0, 0, 0]
  Slice11 : xbsIndex_r4/Slice  nbits=18  boolean_output=off  mode=Lower Bit Location + Width  bit1=0  base1=MSB of Input  bit0=0  base0=LSB of Input  dbl_ovrd=off  block_type=slice
      settings: infoedit="Extracts a given range of bits from each input sample and presents it at the output.  The output type is ordinarily unsigned with binary point at zero, but can be Boolean when the slice is one bit wide.<P><P>Hardware notes: In hardware this block costs nothing."  block_version=10.1.3
  Slice14 : xbsIndex_r4/Slice  nbits=18  boolean_output=off  mode=Lower Bit Location + Width  bit1=0  base1=MSB of Input  bit0=18  base0=LSB of Input  dbl_ovrd=off  block_type=slice
      settings: infoedit="Extracts a given range of bits from each input sample and presents it at the output.  The output type is ordinarily unsigned with binary point at zero, but can be Boolean when the slice is one bit wide.<P><P>Hardware notes: In hardware this block costs nothing."  block_version=10.1.3
  Slice40 : xbsIndex_r4/Slice  nbits=18  boolean_output=off  mode=Lower Bit Location + Width  bit1=0  base1=MSB of Input  bit0=0  base0=LSB of Input  dbl_ovrd=off  block_type=slice
      settings: infoedit="Extracts a given range of bits from each input sample and presents it at the output.  The output type is ordinarily unsigned with binary point at zero, but can be Boolean when the slice is one bit wide.<P><P>Hardware notes: In hardware this block costs nothing."  block_version=10.1.3
  Slice7 : xbsIndex_r4/Slice  nbits=10  boolean_output=off  mode=Lower Bit Location + Width  bit1=0  base1=MSB of Input  bit0=0  base0=LSB of Input  dbl_ovrd=off  block_type=slice
      settings: infoedit="Extracts a given range of bits from each input sample and presents it at the output.  The output type is ordinarily unsigned with binary point at zero, but can be Boolean when the slice is one bit wide.<P><P>Hardware notes: In hardware this block costs nothing."  block_version=10.1.3
  addr : xps_library/software register  Tag=xps:sw_reg  SystemSampleTime=-1  io_dir=From Processor  arith_type=Unsigned  bitwidth=32  bin_pt=0  sample_period=1  gw_name=roachf_1024_bao_EQ_quant2_addr_user_data_out
      link override baopoco_quant0_addr_user_data_out: arith_type=Unsigned  n_bits=32  bin_pt=0  period=1
      link override poco_mod_1024_eq_scale0_user_data_out: arith_type=Unsigned  n_bits=32  bin_pt=0  period=1
      link override poco_mod_1024_no_fd_eq_scale0_user_data_out: arith_type=Unsigned  n_bits=32  bin_pt=0  period=1
      link override poco_mod_eq_scale_user_data_out: arith_type=Unsigned  n_bits=32  bin_pt=0  period=1
      link override poco_red_cd_ld_time_msb_user_data_out: arith_type=Unsigned  n_bits=32  bin_pt=0  period=1
      link override poco_red_fd_ld_time_msb_user_data_out: arith_type=Unsigned  n_bits=32  bin_pt=0  period=1
      link override poco_ref_roach_adc0_cd_ld_time_msb_user_data_out: arith_type=Unsigned  n_bits=32  bin_pt=0  period=1
      link override poco_ref_roach_reduced_adc0_cd_ld_time_msb_user_data_out: arith_type=Unsigned  n_bits=32  bin_pt=0  period=1
      link override poco_roach_red_adc0_cd_ld_time_msb_user_data_out: arith_type=Unsigned  n_bits=32  bin_pt=0  period=1
      link override poco_wide_10_r309_eq_scale0_user_data_out: arith_type=Unsigned  n_bits=32  bin_pt=0  period=1
      link override poco_wide_10_r310_quant0_addr_user_data_out: arith_type=Unsigned  n_bits=32  bin_pt=0  period=1
      link override poco_wide_10_r310_quant3_addr_user_data_out: arith_type=Unsigned  n_bits=32  bin_pt=0  period=1
  eq_store0 : Subsystem  mask{depth_bits=10, n_par=2}
      mask prompts: depth_bits "Number of channels (2^?)"; n_par "Number of parallel streams"
  gain : xps_library/software register  Tag=xps:sw_reg  SystemSampleTime=-1  io_dir=From Processor  arith_type=Unsigned  bitwidth=32  bin_pt=0  sample_period=1  gw_name=roachf_1024_bao_EQ_quant2_gain_user_data_out
      link override baopoco_quant0_gain_user_data_out: arith_type=Unsigned  n_bits=32  bin_pt=0  period=1
      link override poco_mod_1024_eq_scale0_user_data_out: arith_type=Unsigned  n_bits=32  bin_pt=0  period=1
      link override poco_mod_1024_no_fd_eq_scale0_user_data_out: arith_type=Unsigned  n_bits=32  bin_pt=0  period=1
      link override poco_mod_eq_scale_user_data_out: arith_type=Unsigned  n_bits=32  bin_pt=0  period=1
      link override poco_red_cd_ld_time_msb_user_data_out: arith_type=Unsigned  n_bits=32  bin_pt=0  period=1
      link override poco_red_fd_ld_time_msb_user_data_out: arith_type=Unsigned  n_bits=32  bin_pt=0  period=1
      link override poco_ref_roach_adc0_cd_ld_time_msb_user_data_out: arith_type=Unsigned  n_bits=32  bin_pt=0  period=1
      link override poco_ref_roach_reduced_adc0_cd_ld_time_msb_user_data_out: arith_type=Unsigned  n_bits=32  bin_pt=0  period=1
      link override poco_roach_red_adc0_cd_ld_time_msb_user_data_out: arith_type=Unsigned  n_bits=32  bin_pt=0  period=1
      link override poco_wide_10_r309_eq_scale0_user_data_out: arith_type=Unsigned  n_bits=32  bin_pt=0  period=1
      link override poco_wide_10_r310_quant0_gain_user_data_out: arith_type=Unsigned  n_bits=32  bin_pt=0  period=1
      link override poco_wide_10_r310_quant3_gain_user_data_out: arith_type=Unsigned  n_bits=32  bin_pt=0  period=1
  round1 : Subsystem  mask{n_bits=4}
      mask prompts: n_bits "Output Bitwidth"
  round2 : Subsystem  mask{n_bits=4}
      mask prompts: n_bits "Output Bitwidth"
  sync_out : Outport
  clip_out : Outport  Port=2
  dout0 : Outport  Port=3
  dout1 : Outport  Port=4
  wires:
  round1/2(clip) -> Logical5/1
  round2/2(clip) -> Logical5/2
  Constant45/1 -> gain/1
  gain/1 -> Slice40/1
  Slice40/1 -> Delay15/1
  Delay15/1 -> Convert/1
  Delay19/1 -> sync_out/1
  Convert/1 -> eq_store0/2(coeff)
  Slice14/1 -> Convert1/1
  Slice11/1 -> Convert2/1
  eq_store0/1(scale) -> Delay1/1
  Convert1/1 -> round1/2(scale)
  Convert2/1 -> round2/2(scale)
  Constant19/1 -> addr/1
  addr/1 -> Slice7/1
  Slice7/1 -> Delay17/1
  Delay17/1 -> eq_store0/3(coeff_addr)
  Delay18/1 -> Delay3/1
  Delay25/1 -> Delay2/1
  sync/1 -> eq_store0/1(sync), Delay19/1
  din0/1 -> Delay18/1
  round1/1(dout) -> dout0/1
  Logical5/1 -> Delay5/1
  din1/1 -> Delay25/1
  round2/1(dout) -> dout1/1
  Delay1/1 -> Slice11/1, Slice14/1
  Delay2/1 -> round2/1(din)
  Delay3/1 -> round1/1(din)
  Delay5/1 -> clip_out/1
